simulink model "PID_simulation_test"  (R2024b)
settings: Solver=FixedStepAuto  StartTime=0.0  StopTime=1000  FixedStep=0.1  RelTol=1e-3
libraries: simulink_extras x2, slpidlib x1
settings Model: Creator=USER  LastModifiedBy=USER

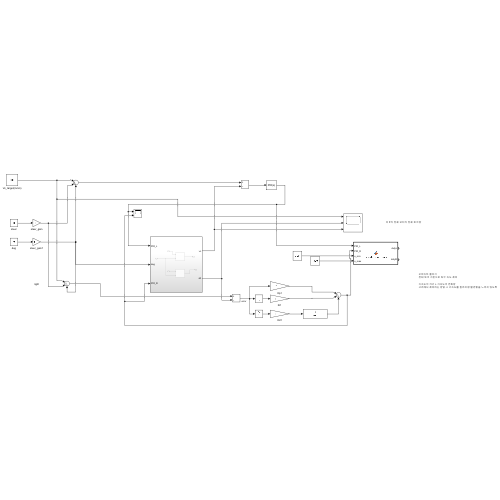
[thumbnail: Simulink's stored preview of the top-level diagram]
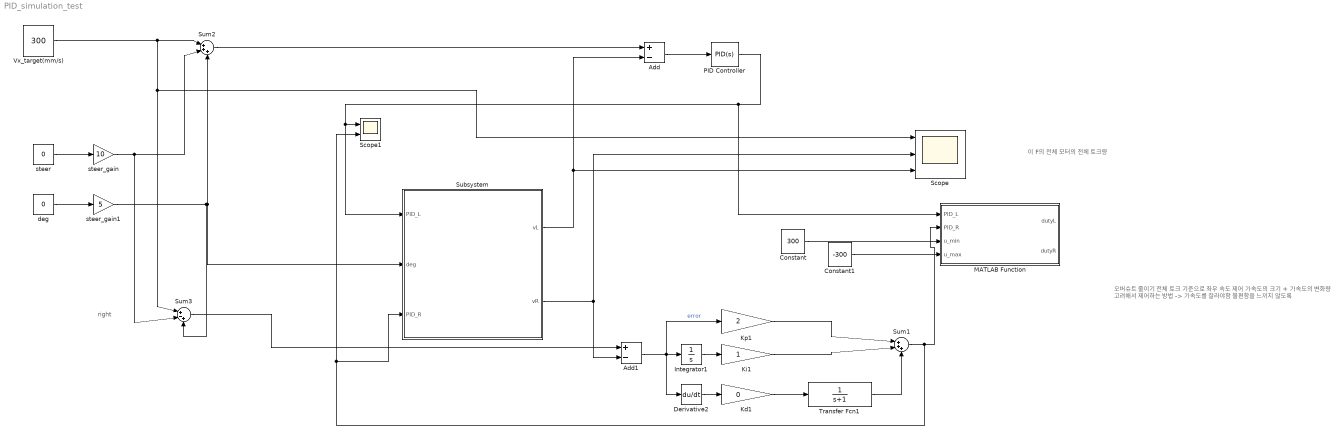
== system PID_simulation_test ==
  note: 이 F의 전체 모터의 전체 토크량
  note: 오버슈트 줄이기
      | 전체 토크 기준으로 좌우 속도 제어
      |
      | 가속도의 크기 + 가속도의 변화량
      | 고려해서 제어하는 방법 -> 가속도를 잘라야함 불편함을 느끼지 않도록
  note: right
  Add : Sum  Inputs=+-
  Add1 : Sum  Inputs=+-
  Constant : Constant  Value=300  OutDataTypeStr=double
  Constant1 : Constant  Value=-300  OutDataTypeStr=double
  Derivative2 : Derivative
  Integrator1 : Integrator
  Kd1 : Gain  Gain=0
  Ki1 : Gain
  Kp1 : Gain  Gain=2
  MATLAB Function : MATLAB Function  TreatAsAtomicUnit=on
  PID Controller : slpidlib/PID Controller  Controller=PID  Form=Parallel  TimeDomain=Continuous-time  UseExternalTs=off  SampleTime=-1  IntegratorMethod=Forward Euler  FilterMethod=Forward Euler  ControllerParametersSource=internal  P=1.50833433531014  I=0.00203455596561696  UseKiTs=off  D=46.0751733553795  UseExternalDerivativeSource=off  N=0.00777088456296687  UseFilter=on  TunerSelectOption=Transfer Function Based (PID Tuner App)  InitialConditionSource=internal  InitialConditionForIntegrator=0  InitialConditionForFilter=0  DifferentiatorICPrevScaledInput=0  ExternalReset=none  TrackingMode=off  Kt=1  LimitOutput=off  SatLimitsSource=internal  UpperSaturationLimit=inf  LowerSaturationLimit=-inf  LinearizeAsGain=on  AntiWindupMode=none  Kb=1  LimitIntegrator=off  UpperIntegratorSaturationLimit=inf  LowerIntegratorSaturationLimit=-inf  POutMin=[]  POutMax=[]  IOutMin=[]  IOutMax=[]  DOutMin=[]  DOutMax=[]  NOutMin=[]  NOutMax=[]  SumOutMin=[]  SumOutMax=[]  SaturationOutMin=[]  SaturationOutMax=[]  PParamMin=[]  PParamMax=[]  IParamMin=[]  IParamMax=[]  DParamMin=[]  DParamMax=[]  NParamMin=[]  NParamMax=[]  KbParamMin=[]  KbParamMax=[]  KtParamMin=[]  KtParamMax=[]  KbOutMin=[]  KbOutMax=[]  KtOutMin=[]  KtOutMax=[]  IntegratorOutMin=[]  IntegratorOutMax=[]  FilterOutMin=[]  FilterOutMax=[]  SumI1OutMin=[]  SumI1OutMax=[]  SumI2OutMin=[]  SumI2OutMax=[]  SumI3OutMin=[]  SumI3OutMax=[]  SumI4OutMin=[]  SumI4OutMax=[]  SumDOutMin=[]  SumDOutMax=[]  DifferentiatorOutMin=[]  DifferentiatorOutMax=[]  FilterDiffOutCoefMin=[]  FilterDiffOutCoefMax=[]  ReciprocalOutMin=[]  ReciprocalOutMax=[]  SumDenOutMin=[]  SumDenOutMax=[]  SumNumOutMin=[]  SumNumOutMax=[]  DivideOutMin=[]  DivideOutMax=[]  UdiffTsProdOutMin=[]  UdiffTsProdOutMax=[]  NTsProdOutMin=[]  NTsProdOutMax=[]  UintegralTsProdOutMin=[]  UintegralTsProdOutMax=[]  UngainTsProdOutMin=[]  UngainTsProdOutMax=[]  ClampingZeroOutDataTypeStr=Inherit: Inherit via back propagation  ClampingZeroOutMin=[]  ClampingZeroOutMax=[]  FilterDenConstantOutDataTypeStr=Inherit: Inherit via back propagation  FilterDenConstantOutMin=[]  FilterDenConstantOutMax=[]  PCopyOutDataTypeStr=Inherit: Inherit via back propagation  PCopyOutMin=[]  PCopyOutMax=[]  NCopyOutDataTypeStr=Inherit: Inherit via back propagation  NCopyOutMin=[]  NCopyOutMax=[]  IntegratorContinuousStateAttributes=''  IntegratorStateMustResolveToSignalObject=off  IntegratorRTWStateStorageClass=Auto  FilterContinuousStateAttributes=''  FilterStateMustResolveToSignalObject=off  FilterRTWStateStorageClass=Auto  ParallelPVariant=InternalParameters  IdealPVariant=Disabled  IVariant=InternalParameters  DVariant=InternalParameters  IntegratorVariant=Continuous  SatVariant=Disabled  AWVariant=Passthrough  PCopyVariant=Disabled  TRVariant=Disabled  FdbkBlocksVariant=Forward  IdealPFdbkVariant=Disabled  SatFdbkVariant=Disabled  DerivativeFilterVariant=ContFilter  NVariant=InternalParameters  NCopyVariant=Disabled  FilterICVariant=InternalICsFilter  IntegratorICVariant=InternalICs  ExternalResetVariant=Disabled  TRSumVariant=Passthrough  SumFdbkVariant=Disabled  SumVariant=Sum_PID  TsampFilterVariant=InternalTs  TsampNgainVariant=Passthrough  TsampIntegralVariant=Disabled_SignalSpec  ExternalSaturationOutDataTypeStr=Inherit: Same as second input  DerivativeSourceVariant=ErrorSignal  PreIntVariant=InternalPreInt
  Scope : Scope  NumInputPorts=3
  Scope1 : Scope  NumInputPorts=2
  Subsystem : Subsystem
  Sum1 : Sum  Inputs=|+++
  Sum2 : Sum  Inputs=|+++
  Sum3 : Sum  Inputs=|+-+
  Transfer Fcn1 : TransferFcn  Denominator=[1 1]
  Vx_target(mm/s) : Constant  Value=300
  deg : Constant  Value=0
  steer : Constant  Value=0
  steer_gain : Gain  Gain=10
  steer_gain1 : Gain  Gain=5
  wires:
  PID Controller/1 -> MATLAB Function/1(PID_L), Subsystem/1(PID_L), Scope1/1
  steer/1 -> steer_gain/1
  Kd1/1 -> Transfer Fcn1/1
  Ki1/1 -> Sum1/2
  Kp1/1 -> Sum1/1
  Derivative2/1 -> Kd1/1
  Integrator1/1 -> Ki1/1
  Sum1/1 -> MATLAB Function/2(PID_R), Scope1/2, Subsystem/3(PID_R)
  Vx_target(mm/s)/1 -> Sum3/1, Scope/1, Sum2/1
  Sum2/1 -> Add/1
  steer_gain/1 -> Sum2/2, Sum3/2
  Sum3/1 -> Add1/1
  Add1/1 -> Derivative2/1, Integrator1/1, Kp1/1  "error"
  deg/1 -> steer_gain1/1
  steer_gain1/1 -> Subsystem/2(deg), Sum2/3, Sum3/3
  Add/1 -> PID Controller/1
  Transfer Fcn1/1 -> Sum1/3
  Subsystem/1(vL) -> Add/2, Scope/3
  Subsystem/2(vR) -> Add1/2, Scope/2
  Constant/1 -> MATLAB Function/3(u_min)
  Constant1/1 -> MATLAB Function/4(u_max)

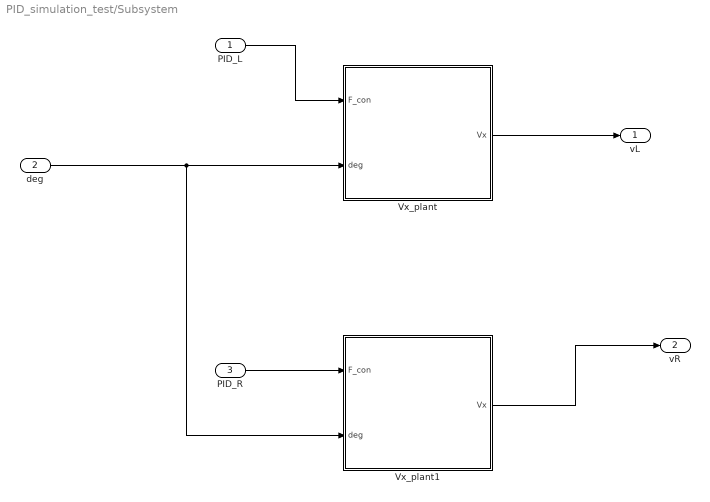
== system PID_simulation_test/Subsystem ==
  PID_L : Inport
  deg : Inport  Port=2
  PID_R : Inport  Port=3
  Vx_plant : Subsystem
  Vx_plant1 : Subsystem
  vL : Outport
  vR : Outport  Port=2
  wires:
  deg/1 -> Vx_plant1/2(deg), Vx_plant/2(deg)
  PID_R/1 -> Vx_plant1/1(F_con)
  Vx_plant1/1(Vx) -> vR/1
  Vx_plant/1(Vx) -> vL/1
  PID_L/1 -> Vx_plant/1(F_con)

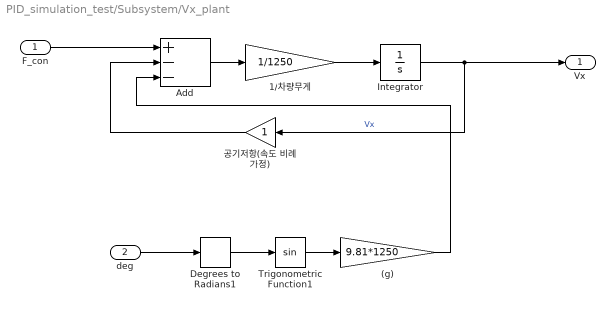
== system PID_simulation_test/Subsystem/Vx_plant ==
  F_con : Inport
  deg : Inport  Port=2
  (g) : Gain  Gain=9.81*1250
  1/차량무게 : Gain  Gain=1/1250
  Add : Sum  Inputs=+--
  Degrees to Radians1 : simulink_extras/Transformations/Degrees to Radians
  Integrator : Integrator
  Trigonometric Function1 : Trigonometry
  공기저항(속도 비례 가정) : Gain
  Vx : Outport
  wires:
  Integrator/1 -> Vx/1, 공기저항(속도 비례 가정)/1  "Vx"
  Add/1 -> 1/차량무게/1
  F_con/1 -> Add/1
  1/차량무게/1 -> Integrator/1
  공기저항(속도 비례 가정)/1 -> Add/2
  Degrees to Radians1/1 -> Trigonometric Function1/1
  Trigonometric Function1/1 -> (g)/1
  deg/1 -> Degrees to Radians1/1
  (g)/1 -> Add/3

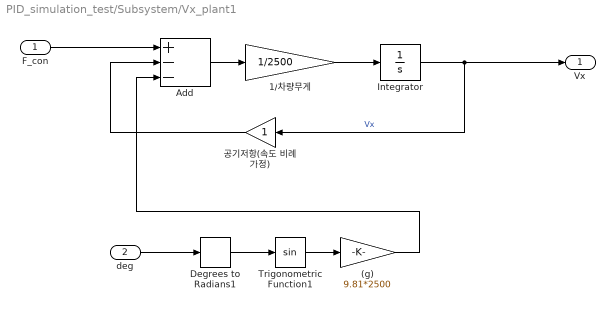
== system PID_simulation_test/Subsystem/Vx_plant1 ==
  F_con : Inport
  deg : Inport  Port=2
  (g) : Gain  Gain=9.81*2500
  1/차량무게 : Gain  Gain=1/2500
  Add : Sum  Inputs=+--
  Degrees to Radians1 : simulink_extras/Transformations/Degrees to Radians
  Integrator : Integrator
  Trigonometric Function1 : Trigonometry
  공기저항(속도 비례 가정) : Gain
  Vx : Outport
  wires:
  (g)/1 -> Add/3
  deg/1 -> Degrees to Radians1/1
  Trigonometric Function1/1 -> (g)/1
  Degrees to Radians1/1 -> Trigonometric Function1/1
  공기저항(속도 비례 가정)/1 -> Add/2
  1/차량무게/1 -> Integrator/1
  F_con/1 -> Add/1
  Add/1 -> 1/차량무게/1
  Integrator/1 -> 공기저항(속도 비례 가정)/1, Vx/1  "Vx"

== matlab function PID_simulation_test/MATLAB Function ==
  data: PID_L input; dutyL output; PID_R input; dutyR output; u_min input; u_max input
function [dutyL, dutyR] = encode_pwm_duty(PID_L, PID_R, u_min, u_max)
% PID_L, PID_R : PID 제어기 출력값 (실수형)
% u_min, u_max : PID 출력 예상 범위 (예: -4050 ~ +4050)

% 매핑 대상 범위
min_duty = -1000;
max_duty = 1000;

%% 매핑 함수 정의
map_to_range = @(u) ((u - u_min) / (u_max - u_min)) * (max_duty - min_duty) + min_duty;

% 매핑 수행
dutyL = round(map_to_range(PID_L));  % 정수로 변환
dutyR = round(map_to_range(PID_R));
